simulink model "controller_dev_sg_HIL"  (R2018b)
settings: configuration reference "Physics" (kept outside this file)
model workspace (MAT data in the model file):
  m = 1000
undefined symbols (not defined in the file or in its folder): C, P_MLOC_NumberOfNoSendFrames, TUMHealthStatus, TUMStateEstimationState, x0_vehiclepose_stm
libraries: speedgoatlib_IO614 x7, xpcrtudplib x7, simulink x6, canmsglib x6, etargetslib x5, xpcutilitieslib x1
settings Model: DataDictionary=controller_dev_sg.sldd  sg_rtwmakecfg_data=_sglibc__IO61X_Library_  PauseTimes=9.280  Creator=wischnewski  LastModifiedBy=ge34qer

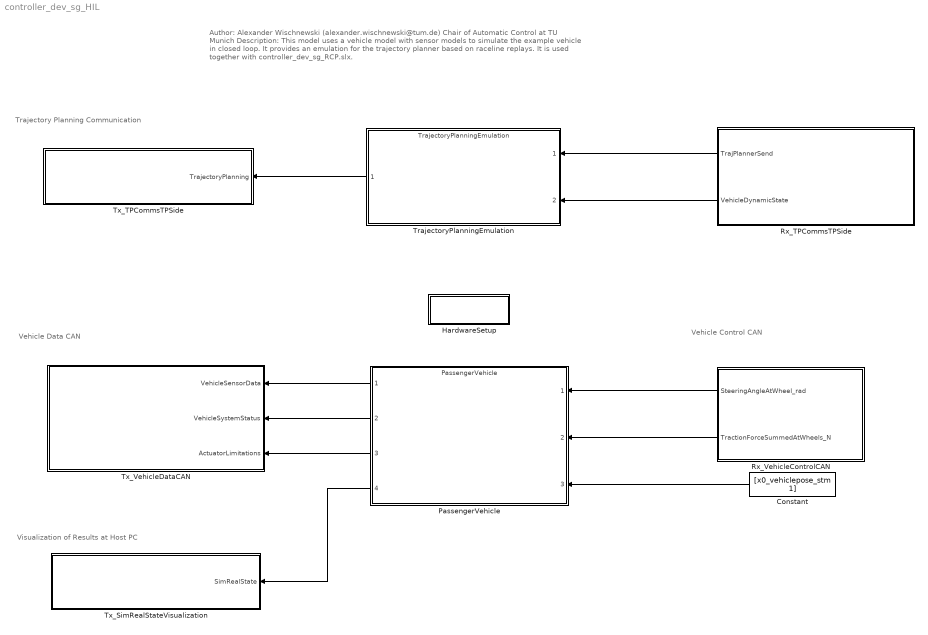
== system controller_dev_sg_HIL ==
  note: Visualization of Results at Host PC
  note: Trajectory Planning Communication
  note: Vehicle Control CAN
  note: Vehicle Data CAN
  note: Author: Alexander Wischnewski (alexander.wischnewski@tum.de)
      | Chair of Automatic Control at TU Munich
      |
      | Description: This model uses a vehicle model with sensor models to simulate the example vehicle in closed loop. It provides an emulation for the trajectory planner based on raceline replays. It is used together with controller_dev_sg_RCP.slx.
  Constant : Constant  Value=[x0_vehiclepose_stm 1]
  HardwareSetup : Subsystem
  PassengerVehicle : ModelReference  ModelNameDialog=PassengerVehicle  SimulationMode=Normal  ModelReferenceVersion=1.774
  Rx_TPCommsTPSide : Subsystem
  Rx_VehicleControlCAN : Subsystem
  TrajectoryPlanningEmulation : ModelReference  ModelNameDialog=TrajectoryPlanningEmulation.slx  SimulationMode=Normal  ModelReferenceVersion=1.722
  Tx_SimRealStateVisualization : Subsystem
  Tx_TPCommsTPSide : Subsystem
  Tx_VehicleDataCAN : Subsystem
  wires:
  PassengerVehicle/4 -> Tx_SimRealStateVisualization/1(SimRealState)
  Rx_TPCommsTPSide/1(TrajPlannerSend) -> TrajectoryPlanningEmulation/1
  TrajectoryPlanningEmulation/1 -> Tx_TPCommsTPSide/1(TrajectoryPlanning)
  Rx_VehicleControlCAN/1(SteeringAngleAtWheel_rad) -> PassengerVehicle/1
  Rx_VehicleControlCAN/2(TractionForceSummedAtWheels_N) -> PassengerVehicle/2
  PassengerVehicle/1 -> Tx_VehicleDataCAN/1(VehicleSensorData)
  PassengerVehicle/2 -> Tx_VehicleDataCAN/2(VehicleSystemStatus)
  PassengerVehicle/3 -> Tx_VehicleDataCAN/3(ActuatorLimitations)
  Rx_TPCommsTPSide/2(VehicleDynamicState) -> TrajectoryPlanningEmulation/2
  Constant/1 -> PassengerVehicle/3

== system controller_dev_sg_HIL/HardwareSetup ==
  CAN & LIN Setup : speedgoatlib_IO614/CAN & LIN Setup  id=1  drLtr=C:  PCISlot=-1  port1=CAN (HS/LS)  port2=CAN (HS)  port3=Disable  port4=Disable  opModeCAN1=Highspeed (HS)  bdrCAN1=1 MBaud  usrBdrCAN1=[5, 1, 13, 2]  stdAccMaskCAN1=[0, 0]  extAccMaskCAN1=[0, 0]  opModeCAN2=Highspeed (HS)  bdrCAN2=1 MBaud  usrBdrCAN2=[5, 1, 13, 2]  stdAccMaskCAN2=[0, 0]  extAccMaskCAN2=[0, 0]  opModeCAN3=Highspeed (HS)  bdrCAN3=1 MBaud  usrBdrCAN3=[5, 1, 13, 2]  stdAccMaskCAN3=[0, 0]  extAccMaskCAN3=[0, 0]  opModeCAN4=Highspeed (HS)  bdrCAN4=1 MBaud  usrBdrCAN4=[5, 1, 13, 2]  stdAccMaskCAN4=[0, 0]  extAccMaskCAN4=[0, 0]  initStruct=[]  termStruct=[]  opModeLIN=Master  bdrLIN=19200  protl=IO614  qtyMod=1  chNo=[1, 2, 3, 4]  ptTypes=[1, 1, 1, 1, 2]  protlHelpIdx=[0, 1, 2, 3, 0]  isFDMod=0  drvLtr=C:  opModeLIN2=Master  bdrLIN2=19200
      settings: SourceProductName=Simulink Real-Time: Speedgoat Library
  "Real-time UDP Configuration " : xpcrtudplib/UDP Configure  Priority=1  IpAddress=10.0.0.2  SubnetMask=255.255.255.0  Gateway=0.0.0.0  PciBus=14  PciSlot=0  PciFunction=0  ID=3  tune=0  disable=off  enableMulticast=off  MulticastIpAddress={}  MulticastMask={}
      settings: SourceProductName=Simulink Real-Time  SourceProductBaseCode=XP

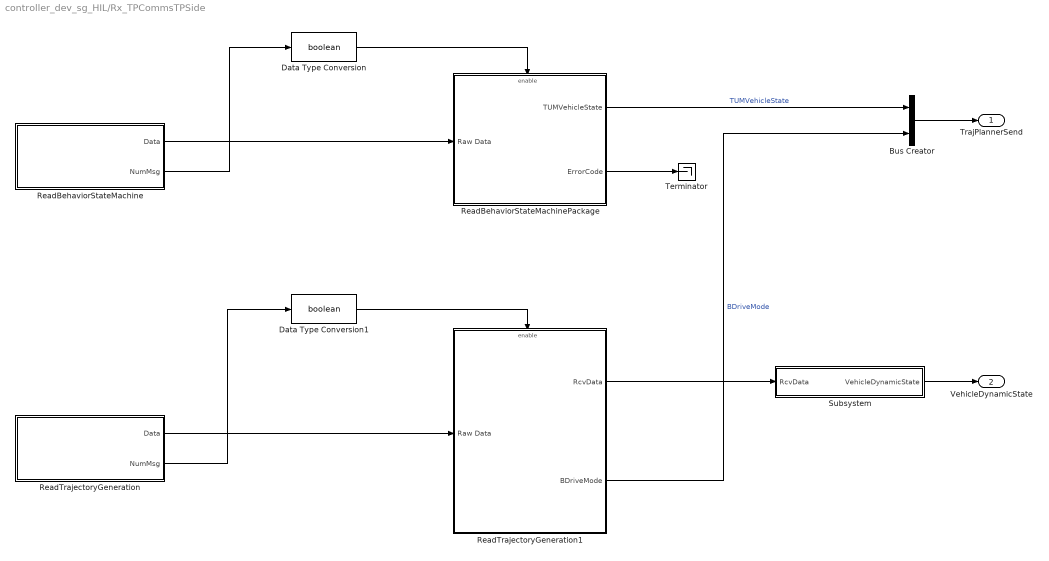
== system controller_dev_sg_HIL/Rx_TPCommsTPSide ==
  Bus Creator : BusCreator  Inputs=2
  Data Type Conversion : DataTypeConversion  OutDataTypeStr=boolean
  Data Type Conversion1 : DataTypeConversion  OutDataTypeStr=boolean
  ReadBehaviorStateMachine : Subsystem  Priority=1000
  ReadBehaviorStateMachinePackage : Subsystem  Priority=1000
  ReadTrajectoryGeneration : Subsystem  Priority=1000
  ReadTrajectoryGeneration1 : Subsystem  Priority=1000
  Subsystem : Subsystem
  Terminator : Terminator
  TrajPlannerSend : Outport  OutDataTypeStr=Bus: TrajPlanner_Send
  VehicleDynamicState : Outport  Port=2  OutDataTypeStr=Bus: VehicleDynamicState
  wires:
  ReadBehaviorStateMachinePackage/1(TUMVehicleState) -> Bus Creator/1  "TUMVehicleState"
  Bus Creator/1 -> TrajPlannerSend/1
  ReadTrajectoryGeneration1/2(BDriveMode) -> Bus Creator/2  "BDriveMode"
  ReadBehaviorStateMachinePackage/2(ErrorCode) -> Terminator/1
  Data Type Conversion/1 -> ReadBehaviorStateMachinePackage/Enable
  Data Type Conversion1/1 -> ReadTrajectoryGeneration1/Enable
  ReadBehaviorStateMachine/2(NumMsg) -> Data Type Conversion/1
  ReadBehaviorStateMachine/1(Data) -> ReadBehaviorStateMachinePackage/1(Raw Data)
  ReadTrajectoryGeneration/1(Data) -> ReadTrajectoryGeneration1/1(Raw Data)
  ReadTrajectoryGeneration/2(NumMsg) -> Data Type Conversion1/1
  Subsystem/1(VehicleDynamicState) -> VehicleDynamicState/1
  ReadTrajectoryGeneration1/1(RcvData) -> Subsystem/1(RcvData)

== system controller_dev_sg_HIL/Rx_VehicleControlCAN ==
  CAN Read : speedgoatlib_IO614/CAN/CAN Read  id=1  sampleTime=-1  portSelection=1  messageType=CAN  protl=IO614  ptIdx=0  isFDMod=0
      settings: SourceProductName=Simulink Real-Time: Speedgoat Library
  CAN Unpack : canmsglib/CAN Unpack  MsgList=(none)  MsgName=CAN Msg  MsgIDType=Standard (11-bit identifier)  MsgIdentifier=24  MsgLength=8  SignalInfo=SteeringAngleAtWheel_rad$0$24$1$1$1$0$0.000001$0$-Inf$Inf$#TractionforceSummedAtWheels_N$24$24$1$1$1$0$0.01$0$-Inf$Inf$#  NSignals=2  IDPort=off  TimestampPort=off  ErrorPort=off  RemotePort=off  LengthPort=off  StatusPort=off  StartBits=str2num('[int32(0);int32(24)]')  SignalSizes=str2num('[int32(24);int32(24)]')  ByteOrders=str2num('[int32(1);int32(1)]')  DataTypes=str2num('[int32(1);int32(1)]')  MultiplexTypes=str2num('[int32(1);int32(1)]')  MultiplexValues=str2num('[double(0);double(0)]')  Factors=str2num('[double(0.000001);double(0.01)]')  Offsets=str2num('[double(0);double(0)]')  Minimums=str2num('[double(-Inf);double(-Inf)]')  Maximums=str2num('[double(Inf);double(Inf)]')  ApplyMinMax=off
      settings: SourceProductName=Simulink Real-Time
  While Iterator : WhileIterator  MaxIters=501  WhileBlockType=do-while
  SteeringAngleAtWheel_rad : Outport
  TractionForceSummedAtWheels_N : Outport  Port=2
  wires:
  CAN Unpack/2 -> TractionForceSummedAtWheels_N/1
  CAN Unpack/1 -> SteeringAngleAtWheel_rad/1
  CAN Read/2 -> CAN Unpack/1
  CAN Read/1 -> While Iterator/1

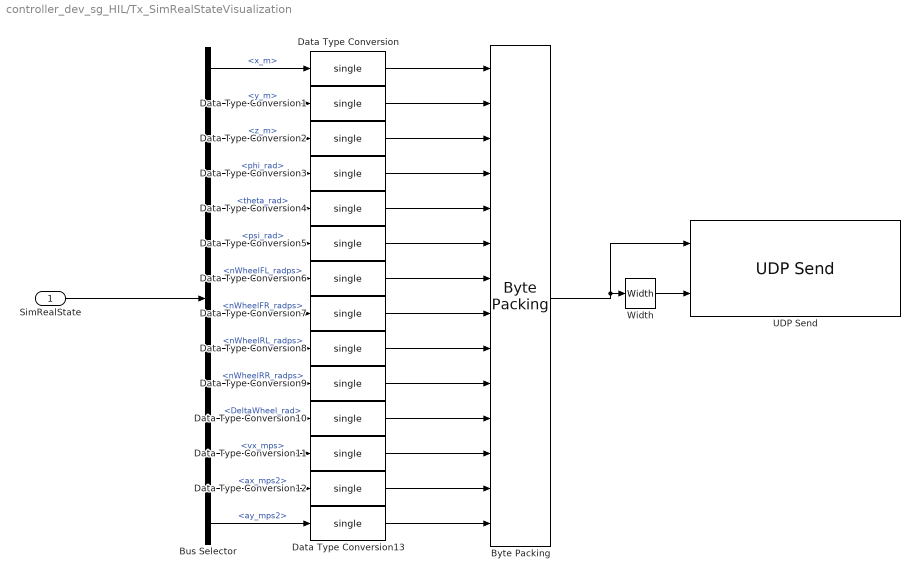
== system controller_dev_sg_HIL/Tx_SimRealStateVisualization ==
  SimRealState : Inport
  Bus Selector : BusSelector  OutputSignals=x_m,y_m,z_m,phi_rad,theta_rad,psi_rad,nWheelFL_radps,nWheelFR_radps,nWheelRL_radps,nWheelRR_radps,DeltaWheel_rad,vx_mps,ax_mps2,ay_mps2
  "Byte Packing " : xpcutilitieslib/Byte Packing   MaskPackedDataType=uint8  MaskUnpackedDataTypes={'single','single','single','single','single','single','single','single','single','single','single','single','single','single'}  MaskAlignment=1
  Data Type Conversion{,1..13} (14 alike) : DataTypeConversion  OutDataTypeStr=single
  UDP Send : xpcrtudplib/UDP Send  ipAddressVal=Use host-target connection  localPort=-1  toAddress=192.168.7.4  toPort=25000  sampleTime=-1
      settings: SourceProductName=Simulink Real-Time  SourceProductBaseCode=XP
  Width : Width
  wires:
  Bus Selector/1 -> Data Type Conversion/1  "<x_m>"
  Bus Selector/2 -> Data Type Conversion1/1  "<y_m>"
  Bus Selector/3 -> Data Type Conversion2/1  "<z_m>"
  Bus Selector/4 -> Data Type Conversion3/1  "<phi_rad>"
  Bus Selector/5 -> Data Type Conversion4/1  "<theta_rad>"
  Bus Selector/6 -> Data Type Conversion5/1  "<psi_rad>"
  Bus Selector/7 -> Data Type Conversion6/1  "<nWheelFL_radps>"
  Bus Selector/8 -> Data Type Conversion7/1  "<nWheelFR_radps>"
  Bus Selector/9 -> Data Type Conversion8/1  "<nWheelRL_radps>"
  Bus Selector/10 -> Data Type Conversion9/1  "<nWheelRR_radps>"
  Bus Selector/11 -> Data Type Conversion10/1  "<DeltaWheel_rad>"
  Data Type Conversion/1 -> "Byte Packing "/1
  Data Type Conversion1/1 -> "Byte Packing "/2
  Data Type Conversion2/1 -> "Byte Packing "/3
  Data Type Conversion3/1 -> "Byte Packing "/4
  Data Type Conversion4/1 -> "Byte Packing "/5
  Data Type Conversion5/1 -> "Byte Packing "/6
  Data Type Conversion6/1 -> "Byte Packing "/7
  Data Type Conversion7/1 -> "Byte Packing "/8
  Data Type Conversion8/1 -> "Byte Packing "/9
  Data Type Conversion9/1 -> "Byte Packing "/10
  Data Type Conversion10/1 -> "Byte Packing "/11
  "Byte Packing "/1 -> UDP Send/1, Width/1
  Width/1 -> UDP Send/2
  Bus Selector/12 -> Data Type Conversion11/1  "<vx_mps>"
  Bus Selector/13 -> Data Type Conversion12/1  "<ax_mps2>"
  Bus Selector/14 -> Data Type Conversion13/1  "<ay_mps2>"
  Data Type Conversion11/1 -> "Byte Packing "/12
  Data Type Conversion12/1 -> "Byte Packing "/13
  Data Type Conversion13/1 -> "Byte Packing "/14
  SimRealState/1 -> Bus Selector/1

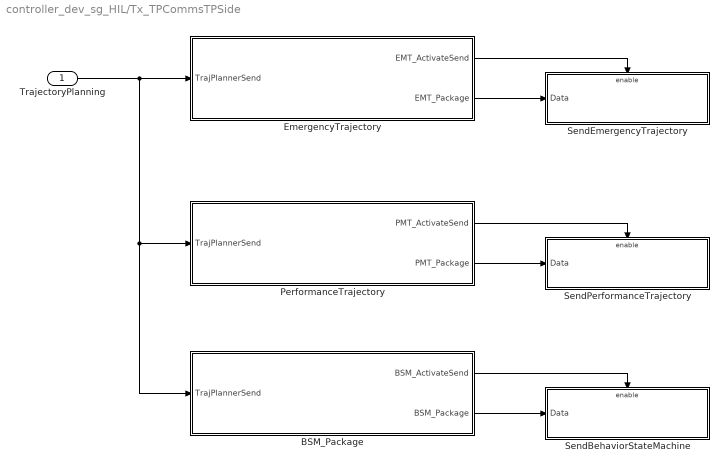
== system controller_dev_sg_HIL/Tx_TPCommsTPSide ==
  TrajectoryPlanning : Inport
  BSM_Package : Subsystem
  EmergencyTrajectory : Subsystem
  PerformanceTrajectory : Subsystem
  SendBehaviorStateMachine : Subsystem
  SendEmergencyTrajectory : Subsystem
  SendPerformanceTrajectory : Subsystem
  wires:
  TrajectoryPlanning/1 -> BSM_Package/1(TrajPlannerSend), PerformanceTrajectory/1(TrajPlannerSend), EmergencyTrajectory/1(TrajPlannerSend)
  EmergencyTrajectory/2(EMT_Package) -> SendEmergencyTrajectory/1(Data)
  PerformanceTrajectory/2(PMT_Package) -> SendPerformanceTrajectory/1(Data)
  BSM_Package/2(BSM_Package) -> SendBehaviorStateMachine/1(Data)
  BSM_Package/1(BSM_ActivateSend) -> SendBehaviorStateMachine/Enable
  PerformanceTrajectory/1(PMT_ActivateSend) -> SendPerformanceTrajectory/Enable
  EmergencyTrajectory/1(EMT_ActivateSend) -> SendEmergencyTrajectory/Enable

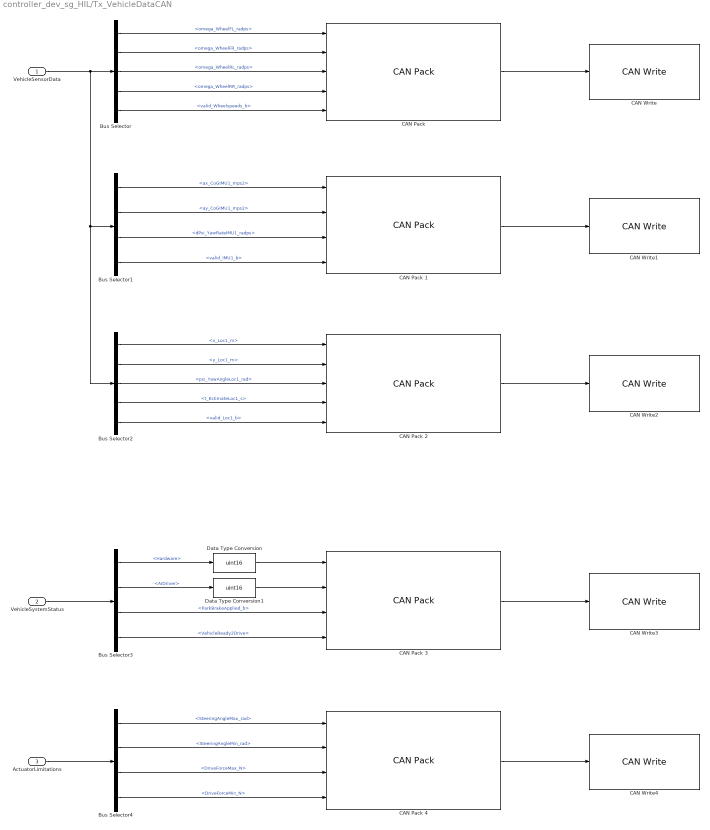
== system controller_dev_sg_HIL/Tx_VehicleDataCAN ==
  VehicleSensorData : Inport
  VehicleSystemStatus : Inport  Port=2
  ActuatorLimitations : Inport  Port=3
  Bus Selector : BusSelector  OutputSignals=omega_WheelFL_radps,omega_WheelFR_radps,omega_WheelRL_radps,omega_WheelRR_radps,valid_Wheelspeeds_b
  Bus Selector1 : BusSelector  OutputSignals=ax_CoGIMU1_mps2,ay_CoGIMU1_mps2,dPsi_YawRateIMU1_radps,valid_IMU1_b
  Bus Selector2 : BusSelector  OutputSignals=x_Loc1_m,y_Loc1_m,psi_YawAngleLoc1_rad,t_EstimateLoc1_s,valid_Loc1_b
  Bus Selector3 : BusSelector  OutputSignals=Hardware,AIDriver,ParkBrakeApplied_b,VehicleReady2Drive
  Bus Selector4 : BusSelector  OutputSignals=SteeringAngleMax_rad,SteeringAngleMin_rad,DriveForceMax_N,DriveForceMin_N
  "CAN Pack " : canmsglib/CAN Pack  MsgList=(none)  MsgName=CAN Msg  MsgIDType=Standard (11-bit identifier)  MsgIdentifier=768  MsgLength=8  SignalInfo=omega_WheelFL_radps$0$15$1$1$1$0$0.1$0$-Inf$Inf$#omega_WheelFR_radps$15$15$1$1$1$0$0.1$0$-Inf$Inf$#omega_WheelRL_radps$30$15$1$1$1$0$0.1$0$-Inf$Inf$#omega_WheelRR_radps$45$15$1$1$1$0$0.1$0$-Inf$Inf$#valid_Wheelspeeds_b$60$4$1$1$1$0$1$0$-Inf$Inf$#  NSignals=5  StartBits=str2num('[int32(0);int32(15);int32(30);int32(45);int32(60)]')  SignalSizes=str2num('[int32(15);int32(15);int32(15);int32(15);int32(4)]')  ByteOrders=str2num('[int32(1);int32(1);int32(1);int32(1);int32(1)]')  DataTypes=str2num('[int32(1);int32(1);int32(1);int32(1);int32(1)]')  MultiplexTypes=str2num('[int32(1);int32(1);int32(1);int32(1);int32(1)]')  MultiplexValues=str2num('[double(0);double(0);double(0);double(0);double(0)]')  Factors=str2num('[double(0.1);double(0.1);double(0.1);double(0.1);double(1)]')  Offsets=str2num('[double(0);double(0);double(0);double(0);double(0)]')  Minimums=str2num('[double(-Inf);double(-Inf);double(-Inf);double(-Inf);double(-Inf)]')  Maximums=str2num('[double(Inf);double(Inf);double(Inf);double(Inf);double(Inf)]')  Remote=off  ApplyMinMax=off  BusOutput=off
      settings: SourceProductName=Simulink Real-Time  DataFormat=manually specified signals
  CAN Pack 1 : canmsglib/CAN Pack  MsgList=(none)  MsgName=CAN Msg  MsgIDType=Standard (11-bit identifier)  MsgIdentifier=48  MsgLength=8  SignalInfo=ax_CoGIMU1_mps2$0$16$1$1$1$0$0.001$0$-Inf$Inf$#ay_CoGIMU1_mps2$16$16$1$1$1$0$0.001$0$-Inf$Inf$#dPsi_YawRateIMU1_radps$32$16$1$1$1$0$0.0001$0$-Inf$Inf$#valid_IMU1_b$48$16$1$1$1$0$1$0$-Inf$Inf$#  NSignals=4  StartBits=str2num('[int32(0);int32(16);int32(32);int32(48)]')  SignalSizes=str2num('[int32(16);int32(16);int32(16);int32(16)]')  ByteOrders=str2num('[int32(1);int32(1);int32(1);int32(1)]')  DataTypes=str2num('[int32(1);int32(1);int32(1);int32(1)]')  MultiplexTypes=str2num('[int32(1);int32(1);int32(1);int32(1)]')  MultiplexValues=str2num('[double(0);double(0);double(0);double(0)]')  Factors=str2num('[double(0.001);double(0.001);double(0.0001);double(1)]')  Offsets=str2num('[double(0);double(0);double(0);double(0)]')  Minimums=str2num('[double(-Inf);double(-Inf);double(-Inf);double(-Inf)]')  Maximums=str2num('[double(Inf);double(Inf);double(Inf);double(Inf)]')  Remote=off  ApplyMinMax=off  BusOutput=off
      settings: SourceProductName=Simulink Real-Time  DataFormat=manually specified signals
  CAN Pack 2 : canmsglib/CAN Pack  MsgList=(none)  MsgName=CAN Msg  MsgIDType=Standard (11-bit identifier)  MsgIdentifier=192  MsgLength=8  SignalInfo=x_Loc1_m$0$15$1$1$1$0$0.05$0$-Inf$Inf$#y_Loc1_m$15$15$1$1$1$0$0.05$0$-Inf$Inf$#psi_YawAngleLoc1_rad$30$15$1$1$1$0$0.001$0$-Inf$Inf$#t_EstimateLoc1_s$45$15$1$1$1$0$0.001$0$-Inf$Inf$#valid_Loc1_b$60$4$1$1$1$0$1$0$-Inf$Inf$#  NSignals=5  StartBits=str2num('[int32(0);int32(15);int32(30);int32(45);int32(60)]')  SignalSizes=str2num('[int32(15);int32(15);int32(15);int32(15);int32(4)]')  ByteOrders=str2num('[int32(1);int32(1);int32(1);int32(1);int32(1)]')  DataTypes=str2num('[int32(1);int32(1);int32(1);int32(1);int32(1)]')  MultiplexTypes=str2num('[int32(1);int32(1);int32(1);int32(1);int32(1)]')  MultiplexValues=str2num('[double(0);double(0);double(0);double(0);double(0)]')  Factors=str2num('[double(0.05);double(0.05);double(0.001);double(0.001);double(1)]')  Offsets=str2num('[double(0);double(0);double(0);double(0);double(0)]')  Minimums=str2num('[double(-Inf);double(-Inf);double(-Inf);double(-Inf);double(-Inf)]')  Maximums=str2num('[double(Inf);double(Inf);double(Inf);double(Inf);double(Inf)]')  Remote=off  ApplyMinMax=off  BusOutput=off
      settings: SourceProductName=Simulink Real-Time  DataFormat=manually specified signals
  CAN Pack 3 : canmsglib/CAN Pack  MsgList=(none)  MsgName=CAN Msg  MsgIDType=Standard (11-bit identifier)  MsgIdentifier=12  MsgLength=8  SignalInfo=Hardware$0$12$1$1$1$0$1$0$-Inf$Inf$#AIDriver$12$12$1$1$1$0$1$0$-Inf$Inf$#ParkBrakeApplied_b$24$12$1$1$1$0$1$0$-Inf$Inf$#VehicleReady2Drive$36$12$1$1$1$0$1$0$-Inf$Inf$#  NSignals=4  StartBits=str2num('[int32(0);int32(12);int32(24);int32(36)]')  SignalSizes=str2num('[int32(12);int32(12);int32(12);int32(12)]')  ByteOrders=str2num('[int32(1);int32(1);int32(1);int32(1)]')  DataTypes=str2num('[int32(1);int32(1);int32(1);int32(1)]')  MultiplexTypes=str2num('[int32(1);int32(1);int32(1);int32(1)]')  MultiplexValues=str2num('[double(0);double(0);double(0);double(0)]')  Factors=str2num('[double(1);double(1);double(1);double(1)]')  Offsets=str2num('[double(0);double(0);double(0);double(0)]')  Minimums=str2num('[double(-Inf);double(-Inf);double(-Inf);double(-Inf)]')  Maximums=str2num('[double(Inf);double(Inf);double(Inf);double(Inf)]')  Remote=off  ApplyMinMax=off  BusOutput=off
      settings: SourceProductName=Simulink Real-Time  DataFormat=manually specified signals
  CAN Pack 4 : canmsglib/CAN Pack  MsgList=(none)  MsgName=CAN Msg  MsgIDType=Standard (11-bit identifier)  MsgIdentifier=170  MsgLength=8  SignalInfo=SteeringAngleMax_rad$0$16$1$1$1$0$0.001$0$-Inf$Inf$#SteeringAngleMin_rad$16$16$1$1$1$0$0.001$0$-Inf$Inf$#DriveForceMax_N$32$16$1$1$1$0$100$0$-Inf$Inf$#DriveForceMin_N$48$16$1$1$1$0$100$0$-Inf$Inf$#  NSignals=4  StartBits=str2num('[int32(0);int32(16);int32(32);int32(48)]')  SignalSizes=str2num('[int32(16);int32(16);int32(16);int32(16)]')  ByteOrders=str2num('[int32(1);int32(1);int32(1);int32(1)]')  DataTypes=str2num('[int32(1);int32(1);int32(1);int32(1)]')  MultiplexTypes=str2num('[int32(1);int32(1);int32(1);int32(1)]')  MultiplexValues=str2num('[double(0);double(0);double(0);double(0)]')  Factors=str2num('[double(0.001);double(0.001);double(100);double(100)]')  Offsets=str2num('[double(0);double(0);double(0);double(0)]')  Minimums=str2num('[double(-Inf);double(-Inf);double(-Inf);double(-Inf)]')  Maximums=str2num('[double(Inf);double(Inf);double(Inf);double(Inf)]')  Remote=off  ApplyMinMax=off  BusOutput=off
      settings: SourceProductName=Simulink Real-Time  DataFormat=manually specified signals
  CAN Write{,1..4} (5 alike) : speedgoatlib_IO614/CAN/CAN Write  id=1  sampleTime=-1  portSelection=2  messageType=CAN  enaStatusPort=off  protl=IO614  ptIdx=1  isFDMod=0
      settings: SourceProductName=Simulink Real-Time: Speedgoat Library
  Data Type Conversion : DataTypeConversion  OutDataTypeStr=uint16
  Data Type Conversion1 : DataTypeConversion  OutDataTypeStr=uint16
  wires:
  Bus Selector/1 -> "CAN Pack "/1  "<omega_WheelFL_radps>"
  Bus Selector/2 -> "CAN Pack "/2  "<omega_WheelFR_radps>"
  Bus Selector/3 -> "CAN Pack "/3  "<omega_WheelRL_radps>"
  Bus Selector/4 -> "CAN Pack "/4  "<omega_WheelRR_radps>"
  Bus Selector/5 -> "CAN Pack "/5  "<valid_Wheelspeeds_b>"
  "CAN Pack "/1 -> CAN Write/1
  Bus Selector1/1 -> CAN Pack 1/1  "<ax_CoGIMU1_mps2>"
  Bus Selector1/2 -> CAN Pack 1/2  "<ay_CoGIMU1_mps2>"
  Bus Selector1/3 -> CAN Pack 1/3  "<dPsi_YawRateIMU1_radps>"
  Bus Selector1/4 -> CAN Pack 1/4  "<valid_IMU1_b>"
  CAN Pack 1/1 -> CAN Write1/1
  CAN Pack 2/1 -> CAN Write2/1
  VehicleSensorData/1 -> Bus Selector2/1, Bus Selector1/1, Bus Selector/1
  Bus Selector2/1 -> CAN Pack 2/1  "<x_Loc1_m>"
  Bus Selector2/2 -> CAN Pack 2/2  "<y_Loc1_m>"
  Bus Selector2/3 -> CAN Pack 2/3  "<psi_YawAngleLoc1_rad>"
  Bus Selector2/5 -> CAN Pack 2/5  "<valid_Loc1_b>"
  VehicleSystemStatus/1 -> Bus Selector3/1
  Bus Selector3/1 -> Data Type Conversion/1  "<Hardware>"
  Bus Selector3/2 -> Data Type Conversion1/1  "<AIDriver>"
  Bus Selector3/3 -> CAN Pack 3/3  "<ParkBrakeApplied_b>"
  Bus Selector3/4 -> CAN Pack 3/4  "<VehicleReady2Drive>"
  CAN Pack 3/1 -> CAN Write3/1
  CAN Pack 4/1 -> CAN Write4/1
  ActuatorLimitations/1 -> Bus Selector4/1
  Bus Selector4/1 -> CAN Pack 4/1  "<SteeringAngleMax_rad>"
  Bus Selector4/2 -> CAN Pack 4/2  "<SteeringAngleMin_rad>"
  Bus Selector4/3 -> CAN Pack 4/3  "<DriveForceMax_N>"
  Bus Selector4/4 -> CAN Pack 4/4  "<DriveForceMin_N>"
  Data Type Conversion/1 -> CAN Pack 3/1
  Data Type Conversion1/1 -> CAN Pack 3/2
  Bus Selector2/4 -> CAN Pack 2/4  "<t_EstimateLoc1_s>"

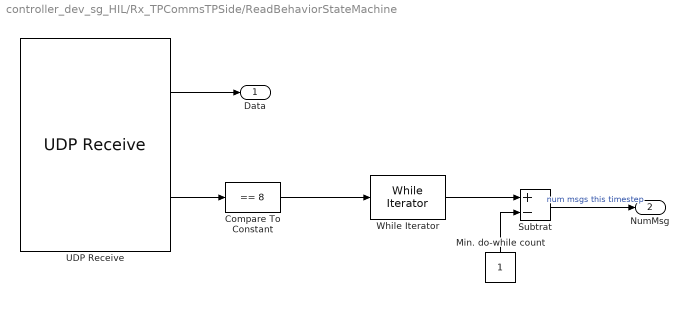
== system controller_dev_sg_HIL/Rx_TPCommsTPSide/ReadBehaviorStateMachine ==
  Compare To Constant : simulink/Logic and Bit Operations/Compare To Constant  relop===  const=8  OutDataTypeStr=boolean
  Min. do-while count : Constant  OutDataTypeStr=int8  SampleTime=-1
  Subtrat : Sum  Inputs=+-
  UDP Receive : xpcrtudplib/UDP Receive  ipAddressVal=10.0.0.2  localPort=BehaviorStatemachineSend_Port  rcvWidth=8  rcvFmAny=off  fmAddress=10.0.0.1  rcvMulticast=off  multicastAddress={}  maxUDPQueue=8  sampleTime=-1
      settings: SourceProductName=Simulink Real-Time
  While Iterator : WhileIterator  WhileBlockType=do-while  ShowIterationPort=on  OutputDataType=int16
  Data : Outport
  NumMsg : Outport  Port=2
  wires:
  Compare To Constant/1 -> While Iterator/1
  UDP Receive/2 -> Compare To Constant/1
  While Iterator/1 -> Subtrat/1
  Min. do-while count/1 -> Subtrat/2
  Subtrat/1 -> NumMsg/1  "num msgs this timestep"
  UDP Receive/1 -> Data/1

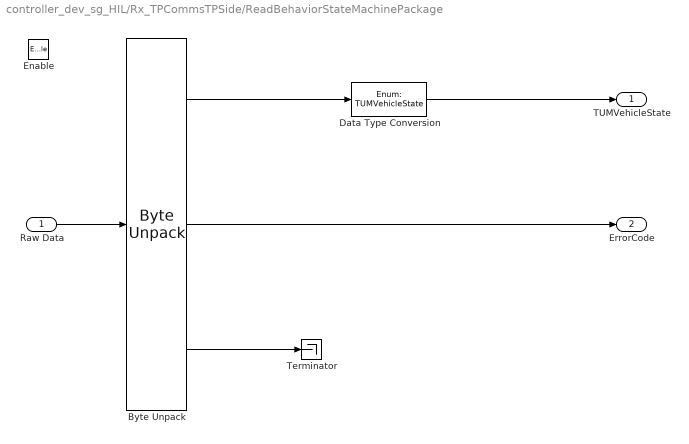
== system controller_dev_sg_HIL/Rx_TPCommsTPSide/ReadBehaviorStateMachinePackage ==
  Raw Data : Inport
  Enable : EnablePort
  Byte Unpack : etargetslib/Byte Unpack  dimensions={[1], [1], [1]}  datatypes={'uint16', 'uint32', 'uint16'}  byteAlign=1
  Data Type Conversion : DataTypeConversion  OutDataTypeStr=Enum: TUMVehicleState  SaturateOnIntegerOverflow=on
  Terminator : Terminator
  TUMVehicleState : Outport
  ErrorCode : Outport  Port=2
  wires:
  Byte Unpack/1 -> Data Type Conversion/1
  Data Type Conversion/1 -> TUMVehicleState/1
  Byte Unpack/2 -> ErrorCode/1
  Raw Data/1 -> Byte Unpack/1
  Byte Unpack/3 -> Terminator/1

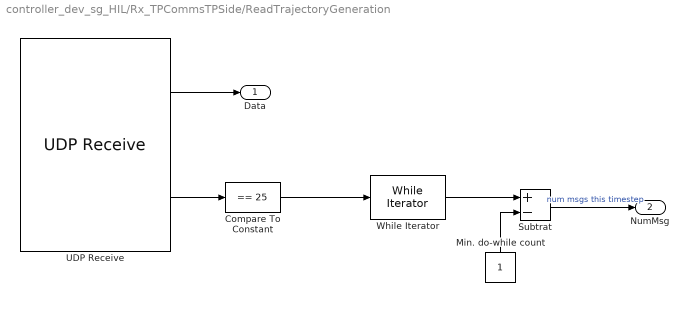
== system controller_dev_sg_HIL/Rx_TPCommsTPSide/ReadTrajectoryGeneration ==
  Compare To Constant : simulink/Logic and Bit Operations/Compare To Constant  relop===  const=25  OutDataTypeStr=boolean
  Min. do-while count : Constant  OutDataTypeStr=int8  SampleTime=-1
  Subtrat : Sum  Inputs=+-
  UDP Receive : xpcrtudplib/UDP Receive  ipAddressVal=10.0.0.2  localPort=TrajectoryGenerationSend_Port  rcvWidth=25  rcvFmAny=off  fmAddress=10.0.0.1  rcvMulticast=off  multicastAddress={}  maxUDPQueue=8  sampleTime=-1
      settings: SourceProductName=Simulink Real-Time
  While Iterator : WhileIterator  WhileBlockType=do-while  ShowIterationPort=on  OutputDataType=int16
  Data : Outport
  NumMsg : Outport  Port=2
  wires:
  Compare To Constant/1 -> While Iterator/1
  UDP Receive/2 -> Compare To Constant/1
  While Iterator/1 -> Subtrat/1
  Min. do-while count/1 -> Subtrat/2
  Subtrat/1 -> NumMsg/1  "num msgs this timestep"
  UDP Receive/1 -> Data/1

== system controller_dev_sg_HIL/Rx_TPCommsTPSide/ReadTrajectoryGeneration1 ==
  Raw Data : Inport
  Enable : EnablePort
  Byte Unpack : etargetslib/Byte Unpack  dimensions={[6], [1]}  datatypes={['single'], 'uint8'}  byteAlign=1
  Data Type Conversion : DataTypeConversion  OutDataTypeStr=double  SaturateOnIntegerOverflow=on
  RcvData : Outport
  BDriveMode : Outport  Port=2
  wires:
  Byte Unpack/2 -> BDriveMode/1
  Raw Data/1 -> Byte Unpack/1
  Byte Unpack/1 -> Data Type Conversion/1
  Data Type Conversion/1 -> RcvData/1

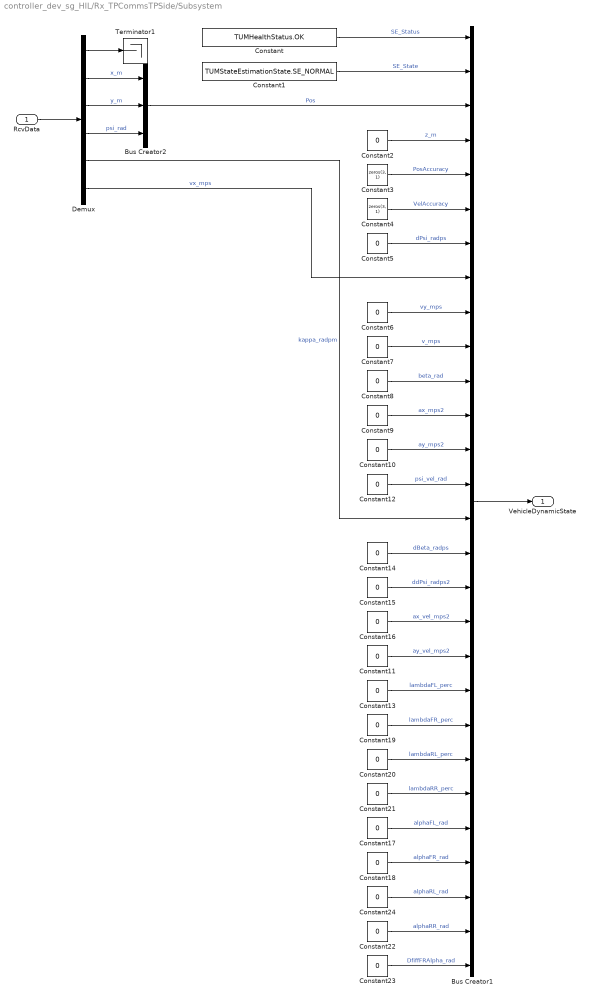
== system controller_dev_sg_HIL/Rx_TPCommsTPSide/Subsystem ==
  RcvData : Inport
  Bus Creator1 : BusCreator  Inputs=28
  Bus Creator2 : BusCreator  Inputs=3  OutDataTypeStr=Bus: CartPos
  Constant : Constant  Value=TUMHealthStatus.OK
  Constant1 : Constant  Value=TUMStateEstimationState.SE_NORMAL
  Constant{2,5..24} (21 alike) : Constant  Value=0
  Constant3 : Constant  Value=zeros(3, 1)
  Constant4 : Constant  Value=zeros(3, 1)
  Demux : Demux  Outputs=6
  Terminator1 : Terminator
  VehicleDynamicState : Outport
  wires:
  Constant/1 -> Bus Creator1/1  "SE_Status"
  Constant1/1 -> Bus Creator1/2  "SE_State"
  Constant24/1 -> Bus Creator1/26  "alphaRL_rad"
  Bus Creator1/1 -> VehicleDynamicState/1
  Constant18/1 -> Bus Creator1/25  "alphaFR_rad"
  Demux/6 -> Bus Creator1/8  "vx_mps"
  Demux/2 -> Bus Creator2/1  "x_m"
  Constant12/1 -> Bus Creator1/14  "psi_vel_rad"
  Constant4/1 -> Bus Creator1/6  "VelAccuracy"
  Bus Creator2/1 -> Bus Creator1/3  "Pos"
  Demux/3 -> Bus Creator2/2  "y_m"
  Constant2/1 -> Bus Creator1/4  "z_m"
  Constant7/1 -> Bus Creator1/10  "v_mps"
  Demux/5 -> Bus Creator1/15  "kappa_radpm"
  Constant17/1 -> Bus Creator1/24  "alphaFL_rad"
  Constant13/1 -> Bus Creator1/20  "lambdaFL_perc"
  Constant15/1 -> Bus Creator1/17  "ddPsi_radps2"
  Constant19/1 -> Bus Creator1/21  "lambdaFR_perc"
  Constant14/1 -> Bus Creator1/16  "dBeta_radps"
  Constant16/1 -> Bus Creator1/18  "ax_vel_mps2"
  Constant6/1 -> Bus Creator1/9  "vy_mps"
  Constant23/1 -> Bus Creator1/28  "DfiffFRAlpha_rad"
  Demux/4 -> Bus Creator2/3  "psi_rad"
  Constant21/1 -> Bus Creator1/23  "lambdaRR_perc"
  Demux/1 -> Terminator1/1
  Constant8/1 -> Bus Creator1/11  "beta_rad"
  Constant3/1 -> Bus Creator1/5  "PosAccuracy"
  Constant5/1 -> Bus Creator1/7  "dPsi_radps"
  Constant22/1 -> Bus Creator1/27  "alphaRR_rad"
  Constant10/1 -> Bus Creator1/13  "ay_mps2"
  RcvData/1 -> Demux/1
  Constant20/1 -> Bus Creator1/22  "lambdaRL_perc"
  Constant9/1 -> Bus Creator1/12  "ax_mps2"
  Constant11/1 -> Bus Creator1/19  "ay_vel_mps2"

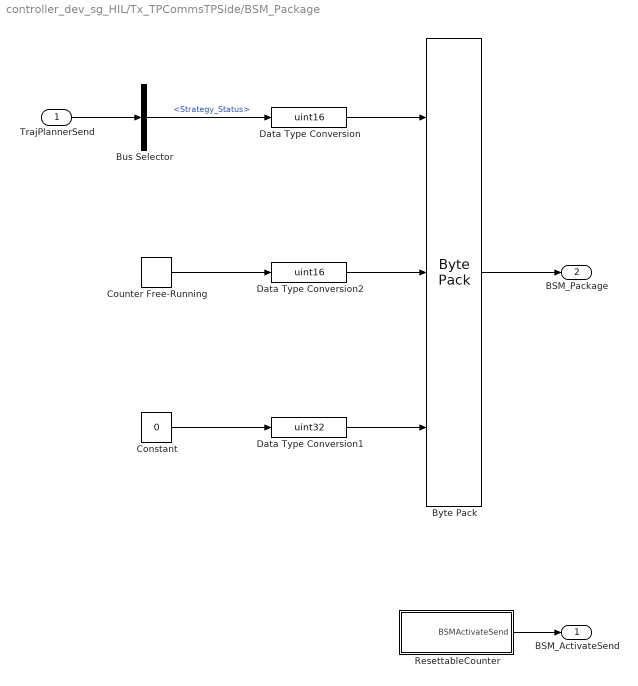
== system controller_dev_sg_HIL/Tx_TPCommsTPSide/BSM_Package ==
  TrajPlannerSend : Inport
  Bus Selector : BusSelector  OutputSignals=Strategy_Status
  Byte Pack : etargetslib/Byte Pack  datatypes={'uint16', 'uint16', 'uint32'}  byteAlign=1
  Constant : Constant  Value=0  SampleTime=-1
  Counter Free-Running : simulink/Sources/Counter Free-Running  NumBits=8  tsamp=-1
  Data Type Conversion : DataTypeConversion  OutDataTypeStr=uint16
  Data Type Conversion1 : DataTypeConversion  OutDataTypeStr=uint32
  Data Type Conversion2 : DataTypeConversion  OutDataTypeStr=uint16
  ResettableCounter : Subsystem
  BSM_ActivateSend : Outport
  BSM_Package : Outport  Port=2
  wires:
  Byte Pack/1 -> BSM_Package/1
  ResettableCounter/1(BSMActivateSend) -> BSM_ActivateSend/1
  TrajPlannerSend/1 -> Bus Selector/1
  Bus Selector/1 -> Data Type Conversion/1  "<Strategy_Status>"
  Data Type Conversion/1 -> Byte Pack/1
  Data Type Conversion1/1 -> Byte Pack/3
  Constant/1 -> Data Type Conversion1/1
  Counter Free-Running/1 -> Data Type Conversion2/1
  Data Type Conversion2/1 -> Byte Pack/2

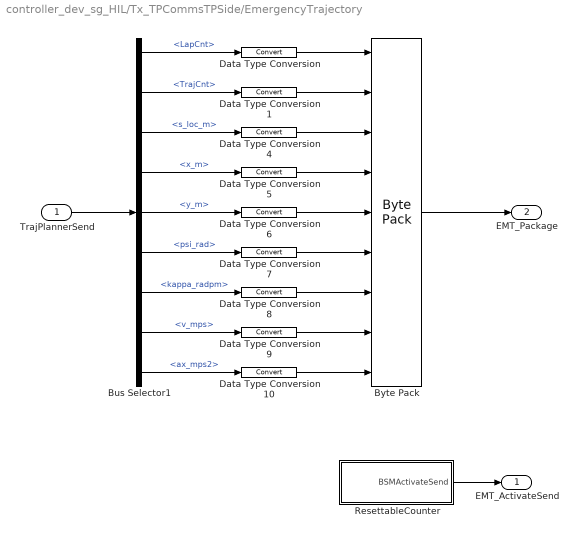
== system controller_dev_sg_HIL/Tx_TPCommsTPSide/EmergencyTrajectory ==
  TrajPlannerSend : Inport
  Bus Selector1 : BusSelector  OutputSignals=EmergencyTrajectory.LapCnt,EmergencyTrajectory.TrajCnt,EmergencyTrajectory.s_loc_m,EmergencyTrajectory.x_m,EmergencyTrajectory.y_m,EmergencyTrajectory.psi_rad,EmergencyTrajectory.kappa_radpm,EmergencyTrajectory.v_mps,EmergencyTrajectory.ax_mps2
  Byte Pack : etargetslib/Byte Pack  datatypes={'uint32', 'uint32', ['single'], ['single'], ['single'], ['single'], ['single'], ['single'], ['single']}  byteAlign=1
  Data Type Conversion{,1,4..10} (9 alike) : DataTypeConversion
  ResettableCounter : Subsystem
  EMT_ActivateSend : Outport
  EMT_Package : Outport  Port=2
  wires:
  Byte Pack/1 -> EMT_Package/1
  ResettableCounter/1(BSMActivateSend) -> EMT_ActivateSend/1
  TrajPlannerSend/1 -> Bus Selector1/1
  Bus Selector1/4 -> Data Type Conversion5/1  "<x_m>"
  Bus Selector1/5 -> Data Type Conversion6/1  "<y_m>"
  Bus Selector1/6 -> Data Type Conversion7/1  "<psi_rad>"
  Bus Selector1/7 -> Data Type Conversion8/1  "<kappa_radpm>"
  Bus Selector1/8 -> Data Type Conversion9/1  "<v_mps>"
  Bus Selector1/9 -> Data Type Conversion10/1  "<ax_mps2>"
  Data Type Conversion/1 -> Byte Pack/1
  Data Type Conversion1/1 -> Byte Pack/2
  Data Type Conversion4/1 -> Byte Pack/3
  Data Type Conversion5/1 -> Byte Pack/4
  Data Type Conversion6/1 -> Byte Pack/5
  Data Type Conversion7/1 -> Byte Pack/6
  Data Type Conversion8/1 -> Byte Pack/7
  Data Type Conversion9/1 -> Byte Pack/8
  Data Type Conversion10/1 -> Byte Pack/9
  Bus Selector1/1 -> Data Type Conversion/1  "<LapCnt>"
  Bus Selector1/2 -> Data Type Conversion1/1  "<TrajCnt>"
  Bus Selector1/3 -> Data Type Conversion4/1  "<s_loc_m>"

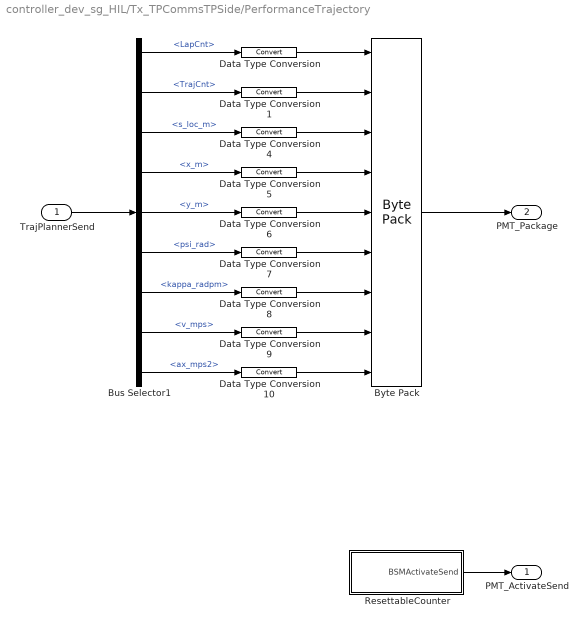
== system controller_dev_sg_HIL/Tx_TPCommsTPSide/PerformanceTrajectory ==
  TrajPlannerSend : Inport
  Bus Selector1 : BusSelector  OutputSignals=PerformanceTrajectory.LapCnt,PerformanceTrajectory.TrajCnt,PerformanceTrajectory.s_loc_m,PerformanceTrajectory.x_m,PerformanceTrajectory.y_m,PerformanceTrajectory.psi_rad,PerformanceTrajectory.kappa_radpm,PerformanceTrajectory.v_mps,PerformanceTrajectory.ax_mps2
  Byte Pack : etargetslib/Byte Pack  datatypes={'uint32', 'uint32', ['single'], ['single'], ['single'], ['single'], ['single'], ['single'], ['single']}  byteAlign=1
  Data Type Conversion{,1,4..10} (9 alike) : DataTypeConversion
  ResettableCounter : Subsystem
  PMT_ActivateSend : Outport
  PMT_Package : Outport  Port=2
  wires:
  ResettableCounter/1(BSMActivateSend) -> PMT_ActivateSend/1
  Bus Selector1/1 -> Data Type Conversion/1  "<LapCnt>"
  Data Type Conversion4/1 -> Byte Pack/3
  Data Type Conversion9/1 -> Byte Pack/8
  Data Type Conversion10/1 -> Byte Pack/9
  Data Type Conversion8/1 -> Byte Pack/7
  Data Type Conversion6/1 -> Byte Pack/5
  Data Type Conversion5/1 -> Byte Pack/4
  Bus Selector1/2 -> Data Type Conversion1/1  "<TrajCnt>"
  Bus Selector1/5 -> Data Type Conversion6/1  "<y_m>"
  Bus Selector1/3 -> Data Type Conversion4/1  "<s_loc_m>"
  Bus Selector1/9 -> Data Type Conversion10/1  "<ax_mps2>"
  Bus Selector1/8 -> Data Type Conversion9/1  "<v_mps>"
  Data Type Conversion7/1 -> Byte Pack/6
  TrajPlannerSend/1 -> Bus Selector1/1
  Data Type Conversion/1 -> Byte Pack/1
  Byte Pack/1 -> PMT_Package/1
  Bus Selector1/6 -> Data Type Conversion7/1  "<psi_rad>"
  Bus Selector1/4 -> Data Type Conversion5/1  "<x_m>"
  Data Type Conversion1/1 -> Byte Pack/2
  Bus Selector1/7 -> Data Type Conversion8/1  "<kappa_radpm>"

== system controller_dev_sg_HIL/Tx_TPCommsTPSide/SendBehaviorStateMachine ==
  Data : Inport
  Enable : EnablePort
  "Send " : xpcrtudplib/UDP Send  ipAddressVal=10.0.0.2  localPort=-1  toAddress=10.0.0.1  toPort=BehaviorStatemachineRcv_Port  sampleTime=-1
      settings: SourceProductName=Simulink Real-Time  SourceProductBaseCode=XP
  Width : Width
  wires:
  Width/1 -> "Send "/2
  Data/1 -> Width/1, "Send "/1

== system controller_dev_sg_HIL/Tx_TPCommsTPSide/SendEmergencyTrajectory ==
  Data : Inport
  Enable : EnablePort
  "Send " : xpcrtudplib/UDP Send  ipAddressVal=10.0.0.2  localPort=-1  toAddress=10.0.0.1  toPort=EmergencyPathRcv_Port  sampleTime=-1
      settings: SourceProductName=Simulink Real-Time  SourceProductBaseCode=XP
  Width : Width
  wires:
  Width/1 -> "Send "/2
  Data/1 -> Width/1, "Send "/1

== system controller_dev_sg_HIL/Tx_TPCommsTPSide/SendPerformanceTrajectory ==
  Data : Inport
  Enable : EnablePort
  "Send " : xpcrtudplib/UDP Send  ipAddressVal=10.0.0.2  localPort=-1  toAddress=10.0.0.1  toPort=PerformanceTrajectoryRcv_Port  sampleTime=-1
      settings: SourceProductName=Simulink Real-Time  SourceProductBaseCode=XP
  Width : Width
  wires:
  Width/1 -> "Send "/2
  Data/1 -> Width/1, "Send "/1

== system controller_dev_sg_HIL/Tx_TPCommsTPSide/BSM_Package/ResettableCounter ==
  Compare To Constant : simulink/Logic and Bit Operations/Compare To Constant  relop=>=  const=5  OutDataTypeStr=boolean
  Constant : Constant
  Constant1 : Constant  Value=0
  Sum : Sum  Inputs=|++
  Switch : Switch  Criteria=u2 ~= 0  Threshold=P_MLOC_NumberOfNoSendFrames
  Unit Delay : UnitDelay  SampleTime=-1
  BSMActivateSend : Outport
  wires:
  Unit Delay/1 -> Compare To Constant/1, Sum/2
  Compare To Constant/1 -> BSMActivateSend/1, Switch/2
  Switch/1 -> Unit Delay/1
  Constant/1 -> Sum/1
  Constant1/1 -> Switch/1
  Sum/1 -> Switch/3

== system controller_dev_sg_HIL/Tx_TPCommsTPSide/EmergencyTrajectory/ResettableCounter ==
  Compare To Constant : simulink/Logic and Bit Operations/Compare To Constant  relop=>=  const=5  OutDataTypeStr=boolean
  Constant : Constant  SampleTime=-1
  Constant1 : Constant  Value=0  SampleTime=-1
  Sum : Sum  Inputs=|++
  Switch : Switch  Criteria=u2 ~= 0  Threshold=P_MLOC_NumberOfNoSendFrames
  Unit Delay : UnitDelay  SampleTime=-1
  BSMActivateSend : Outport
  wires:
  Unit Delay/1 -> Compare To Constant/1, Sum/2
  Compare To Constant/1 -> BSMActivateSend/1, Switch/2
  Switch/1 -> Unit Delay/1
  Constant/1 -> Sum/1
  Constant1/1 -> Switch/1
  Sum/1 -> Switch/3

== system controller_dev_sg_HIL/Tx_TPCommsTPSide/PerformanceTrajectory/ResettableCounter ==
  Compare To Constant : simulink/Logic and Bit Operations/Compare To Constant  relop=>=  const=5  OutDataTypeStr=boolean
  Constant : Constant  SampleTime=-1
  Constant1 : Constant  Value=0  SampleTime=-1
  Sum : Sum  Inputs=|++
  Switch : Switch  Criteria=u2 ~= 0  Threshold=P_MLOC_NumberOfNoSendFrames
  Unit Delay : UnitDelay  SampleTime=-1
  BSMActivateSend : Outport
  wires:
  Unit Delay/1 -> Compare To Constant/1, Sum/2
  Compare To Constant/1 -> BSMActivateSend/1, Switch/2
  Switch/1 -> Unit Delay/1
  Constant/1 -> Sum/1
  Constant1/1 -> Switch/1
  Sum/1 -> Switch/3
